simulink model "modelo_Parcial2_Garcia_Tomas_14077"  (R2018a)
settings: Solver=ode45  StartTime=0.0  StopTime=200  MaxStep=.1  RelTol=1e-3
undefined symbols (not defined in the file): c, m, magnitud_pulso_perturbacion, R, tiempo_pulso_perturbacion
libraries: simulink x3
settings Model: LastModifiedBy=tomas
settings DataIOCC: ReturnWorkspaceOutputs=on
settings DebuggingCC: UnconnectedInputMsg=none  UnconnectedOutputMsg=none  UnconnectedLineMsg=none
settings ModelReferenceCC: UpdateModelReferenceTargets=IfOutOfDate  EnableRefExpFcnMdlSchedulingChecks=off
settings SFSimCC: SimUseLocalCustomCode=on
settings RTWCC: Description=Generic Real-Time Target  RTWUseLocalCustomCode=on

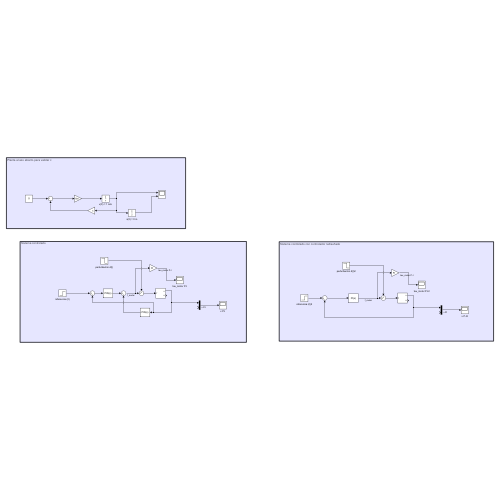
[thumbnail: Simulink's stored preview of the top-level diagram]
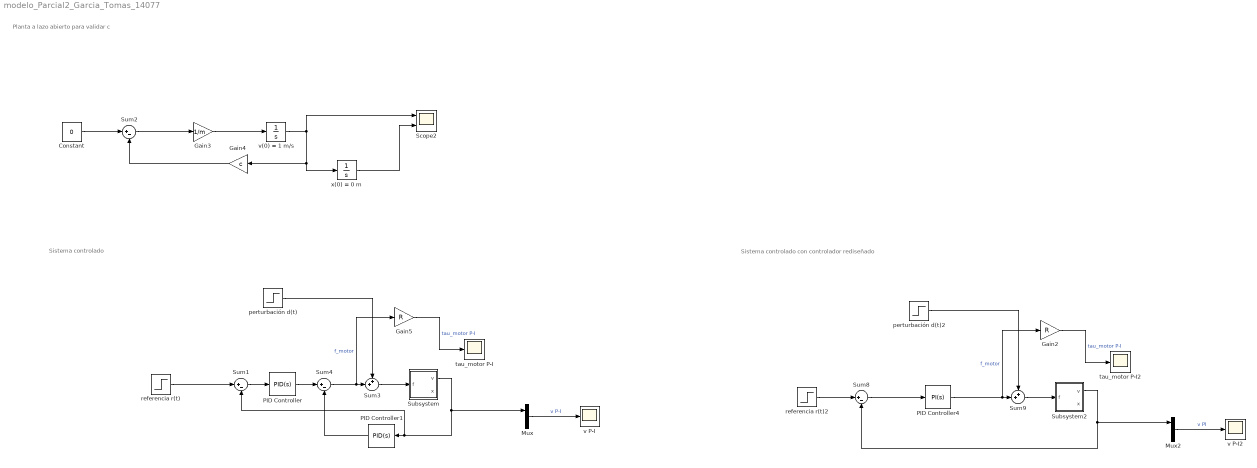
== system modelo_Parcial2_Garcia_Tomas_14077 ==
  note: Sistema controlado con controlador rediseñado
  note: Sistema controlado
  note: Planta a lazo abierto para validar c
  Constant : Constant  Value=0
  Gain2 : Gain  Gain=R
  Gain3 : Gain  Gain=1/m
  Gain4 : Gain  Gain=c
  Gain5 : Gain  Gain=R
  Mux : Mux  Inputs=2
  Mux2 : Mux  Inputs=2
  PID Controller : simulink/Continuous/PID Controller  Controller=PID  Form=Parallel  TimeDomain=Continuous-time  SampleTime=-1  IntegratorMethod=Forward Euler  ControllerParametersSource=internal  P=0  I=500  D=0  N=100  UseFilter=on  TunerSelectOption=Transfer Function Based (PID Tuner App)  InitialConditionSource=internal  InitialConditionForIntegrator=0  InitialConditionForFilter=0  DifferentiatorICPrevScaledInput=0  ExternalReset=none  TrackingMode=off  Kt=1  LimitOutput=off  UpperSaturationLimit=inf  LowerSaturationLimit=-inf  LinearizeAsGain=on  AntiWindupMode=none  Kb=1  POutMin=[]  POutMax=[]  IOutMin=[]  IOutMax=[]  DOutMin=[]  DOutMax=[]  NOutMin=[]  NOutMax=[]  SumOutMin=[]  SumOutMax=[]  SaturationOutMin=[]  SaturationOutMax=[]  PParamMin=[]  PParamMax=[]  IParamMin=[]  IParamMax=[]  DParamMin=[]  DParamMax=[]  NParamMin=[]  NParamMax=[]  KbParamMin=[]  KbParamMax=[]  KtParamMin=[]  KtParamMax=[]  KbOutMin=[]  KbOutMax=[]  KtOutMin=[]  KtOutMax=[]  IntegratorOutMin=[]  IntegratorOutMax=[]  FilterOutMin=[]  FilterOutMax=[]  SumI1OutMin=[]  SumI1OutMax=[]  SumI2OutMin=[]  SumI2OutMax=[]  SumI3OutMin=[]  SumI3OutMax=[]  SumDOutMin=[]  SumDOutMax=[]  DifferentiatorOutMin=[]  DifferentiatorOutMax=[]  FilterDiffOutCoefMin=[]  FilterDiffOutCoefMax=[]  ReciprocalOutMin=[]  ReciprocalOutMax=[]  SumDenOutMin=[]  SumDenOutMax=[]  SumNumOutMin=[]  SumNumOutMax=[]  DivideOutMin=[]  DivideOutMax=[]  IntegratorContinuousStateAttributes=''  IntegratorStateMustResolveToSignalObject=off  IntegratorRTWStateStorageClass=Auto  FilterContinuousStateAttributes=''  FilterStateMustResolveToSignalObject=off  FilterRTWStateStorageClass=Auto
  PID Controller1 : simulink/Continuous/PID Controller  Controller=PID  Form=Parallel  TimeDomain=Continuous-time  SampleTime=-1  IntegratorMethod=Forward Euler  ControllerParametersSource=internal  P=2000  I=0  D=0  N=100  UseFilter=on  TunerSelectOption=Transfer Function Based (PID Tuner App)  InitialConditionSource=internal  InitialConditionForIntegrator=0  InitialConditionForFilter=0  DifferentiatorICPrevScaledInput=0  ExternalReset=none  TrackingMode=off  Kt=1  LimitOutput=off  UpperSaturationLimit=inf  LowerSaturationLimit=-inf  LinearizeAsGain=on  AntiWindupMode=none  Kb=1  POutMin=[]  POutMax=[]  IOutMin=[]  IOutMax=[]  DOutMin=[]  DOutMax=[]  NOutMin=[]  NOutMax=[]  SumOutMin=[]  SumOutMax=[]  SaturationOutMin=[]  SaturationOutMax=[]  PParamMin=[]  PParamMax=[]  IParamMin=[]  IParamMax=[]  DParamMin=[]  DParamMax=[]  NParamMin=[]  NParamMax=[]  KbParamMin=[]  KbParamMax=[]  KtParamMin=[]  KtParamMax=[]  KbOutMin=[]  KbOutMax=[]  KtOutMin=[]  KtOutMax=[]  IntegratorOutMin=[]  IntegratorOutMax=[]  FilterOutMin=[]  FilterOutMax=[]  SumI1OutMin=[]  SumI1OutMax=[]  SumI2OutMin=[]  SumI2OutMax=[]  SumI3OutMin=[]  SumI3OutMax=[]  SumDOutMin=[]  SumDOutMax=[]  DifferentiatorOutMin=[]  DifferentiatorOutMax=[]  FilterDiffOutCoefMin=[]  FilterDiffOutCoefMax=[]  ReciprocalOutMin=[]  ReciprocalOutMax=[]  SumDenOutMin=[]  SumDenOutMax=[]  SumNumOutMin=[]  SumNumOutMax=[]  DivideOutMin=[]  DivideOutMax=[]  IntegratorContinuousStateAttributes=''  IntegratorStateMustResolveToSignalObject=off  IntegratorRTWStateStorageClass=Auto  FilterContinuousStateAttributes=''  FilterStateMustResolveToSignalObject=off  FilterRTWStateStorageClass=Auto
  PID Controller4 : simulink/Continuous/PID Controller  Controller=PI  Form=Parallel  TimeDomain=Continuous-time  SampleTime=-1  IntegratorMethod=Forward Euler  ControllerParametersSource=internal  P=93  I=336.1  D=0  N=100  UseFilter=on  TunerSelectOption=Transfer Function Based (PID Tuner App)  InitialConditionSource=internal  InitialConditionForIntegrator=0  InitialConditionForFilter=0  DifferentiatorICPrevScaledInput=0  ExternalReset=none  TrackingMode=off  Kt=1  LimitOutput=off  UpperSaturationLimit=inf  LowerSaturationLimit=-inf  LinearizeAsGain=on  AntiWindupMode=none  Kb=1  POutMin=[]  POutMax=[]  IOutMin=[]  IOutMax=[]  DOutMin=[]  DOutMax=[]  NOutMin=[]  NOutMax=[]  SumOutMin=[]  SumOutMax=[]  SaturationOutMin=[]  SaturationOutMax=[]  PParamMin=[]  PParamMax=[]  IParamMin=[]  IParamMax=[]  DParamMin=[]  DParamMax=[]  NParamMin=[]  NParamMax=[]  KbParamMin=[]  KbParamMax=[]  KtParamMin=[]  KtParamMax=[]  KbOutMin=[]  KbOutMax=[]  KtOutMin=[]  KtOutMax=[]  IntegratorOutMin=[]  IntegratorOutMax=[]  FilterOutMin=[]  FilterOutMax=[]  SumI1OutMin=[]  SumI1OutMax=[]  SumI2OutMin=[]  SumI2OutMax=[]  SumI3OutMin=[]  SumI3OutMax=[]  SumDOutMin=[]  SumDOutMax=[]  DifferentiatorOutMin=[]  DifferentiatorOutMax=[]  FilterDiffOutCoefMin=[]  FilterDiffOutCoefMax=[]  ReciprocalOutMin=[]  ReciprocalOutMax=[]  SumDenOutMin=[]  SumDenOutMax=[]  SumNumOutMin=[]  SumNumOutMax=[]  DivideOutMin=[]  DivideOutMax=[]  IntegratorContinuousStateAttributes=''  IntegratorStateMustResolveToSignalObject=off  IntegratorRTWStateStorageClass=Auto  FilterContinuousStateAttributes=''  FilterStateMustResolveToSignalObject=off  FilterRTWStateStorageClass=Auto
  Scope2 : Scope  NumInputPorts=2
  Subsystem : Subsystem
  Subsystem2 : Subsystem
  Sum{1..2,4,8} (4 alike) : Sum  Inputs=|+-
  Sum3 : Sum  Inputs=++|
  Sum9 : Sum  Inputs=++|
  perturbación d(t) : Step  Time=tiempo_pulso_perturbacion  After=-magnitud_pulso_perturbacion  SampleTime=0
  perturbación d(t)2 : Step  Time=tiempo_pulso_perturbacion  After=-magnitud_pulso_perturbacion  SampleTime=0
  referencia r(t) : Step  Time=0  SampleTime=0
  referencia r(t)2 : Step  Time=0  SampleTime=0
  tau_motor P-I : Scope
  tau_motor P-I2 : Scope
  v P-I : Scope
  v P-I2 : Scope
  v(0) = 1 m/s : Integrator  InitialCondition=1
  x(0) = 0 m : Integrator
  wires:
  Sum3/1 -> Subsystem/1(f)
  Sum4/1 -> Gain5/1, Sum3/2  "f_motor"
  PID Controller1/1 -> Sum4/2
  PID Controller/1 -> Sum4/1
  Sum1/1 -> PID Controller/1
  referencia r(t)/1 -> Sum1/1
  Subsystem/1(v) -> Mux/1, Sum1/2, PID Controller1/1
  Sum2/1 -> Gain3/1
  Gain3/1 -> v(0) = 1 m/s/1
  v(0) = 1 m/s/1 -> Scope2/1, x(0) = 0 m/1, Gain4/1
  Gain4/1 -> Sum2/2
  Constant/1 -> Sum2/1
  x(0) = 0 m/1 -> Scope2/2
  Mux/1 -> v P-I/1  "v P-I"
  Gain5/1 -> tau_motor P-I/1  "tau_motor P-I"
  perturbación d(t)/1 -> Sum3/1
  Sum8/1 -> PID Controller4/1
  Sum9/1 -> Subsystem2/1(f)
  PID Controller4/1 -> Gain2/1, Sum9/2  "f_motor"
  Mux2/1 -> v P-I2/1  "v PI"
  Subsystem2/1(v) -> Mux2/1, Sum8/2
  Gain2/1 -> tau_motor P-I2/1  "tau_motor P-I"
  referencia r(t)2/1 -> Sum8/1
  perturbación d(t)2/1 -> Sum9/1

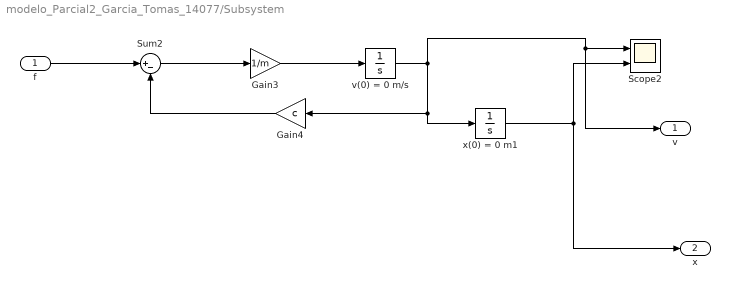
== system modelo_Parcial2_Garcia_Tomas_14077/Subsystem ==
  f : Inport
  Gain3 : Gain  Gain=1/m
  Gain4 : Gain  Gain=c
  Scope2 : Scope  NumInputPorts=2
  Sum2 : Sum  Inputs=|+-
  v(0) = 0 m/s : Integrator
  x(0) = 0 m1 : Integrator
  v : Outport
  x : Outport  Port=2
  wires:
  Gain3/1 -> v(0) = 0 m/s/1
  Sum2/1 -> Gain3/1
  x(0) = 0 m1/1 -> x/1, Scope2/2
  Gain4/1 -> Sum2/2
  v(0) = 0 m/s/1 -> v/1, Scope2/1, x(0) = 0 m1/1, Gain4/1
  f/1 -> Sum2/1

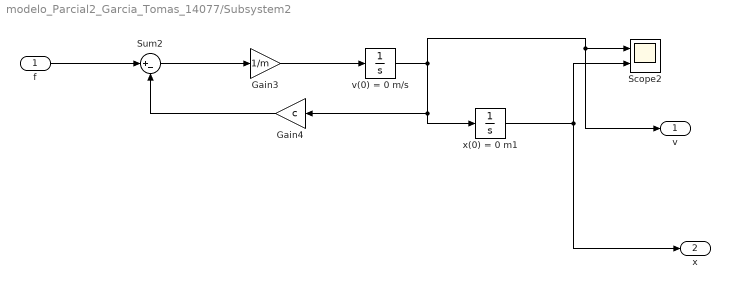
== system modelo_Parcial2_Garcia_Tomas_14077/Subsystem2 ==
  f : Inport
  Gain3 : Gain  Gain=1/m
  Gain4 : Gain  Gain=c
  Scope2 : Scope  NumInputPorts=2
  Sum2 : Sum  Inputs=|+-
  v(0) = 0 m/s : Integrator
  x(0) = 0 m1 : Integrator
  v : Outport
  x : Outport  Port=2
  wires:
  Gain3/1 -> v(0) = 0 m/s/1
  Sum2/1 -> Gain3/1
  x(0) = 0 m1/1 -> x/1, Scope2/2
  Gain4/1 -> Sum2/2
  v(0) = 0 m/s/1 -> v/1, Scope2/1, x(0) = 0 m1/1, Gain4/1
  f/1 -> Sum2/1
